simulink model "modle"  (R2017b)
settings: Solver=VariableStepAuto  StartTime=0.0  StopTime=10.0  RelTol=1e-3
values from neighbouring files (symbols this model uses):
  g = 9.81    [mode.m]
undefined symbols (not defined in the file or in its folder): b, K, L, m
settings Model: Creator=Usuario  LastModifiedBy=Usuario

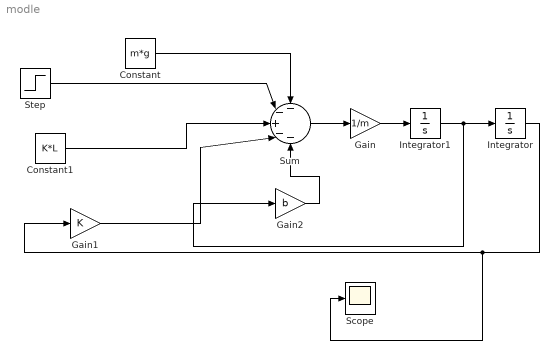
== system modle ==
  Constant : Constant  Value=m*g
  Constant1 : Constant  Value=K*L
  Gain : Gain  Gain=1/m
  Gain1 : Gain  Gain=K
  Gain2 : Gain  Gain=b
  Integrator : Integrator
  Integrator1 : Integrator
  Scope : Scope
  Step : Step  SampleTime=0
  Sum : Sum  Inputs=--+--
  wires:
  Constant/1 -> Sum/1
  Integrator1/1 -> Gain2/1, Integrator/1
  Sum/1 -> Gain/1
  Gain/1 -> Integrator1/1
  Step/1 -> Sum/2
  Constant1/1 -> Sum/3
  Gain1/1 -> Sum/4
  Integrator/1 -> Scope/1, Gain1/1
  Gain2/1 -> Sum/5
